simulink model "Lab4"  (R2025a)
settings: Solver=VariableStepAuto  StartTime=0.0  StopTime=20  RelTol=1e-3
settings Model: Creator=andrei  LastModifiedBy=andrei

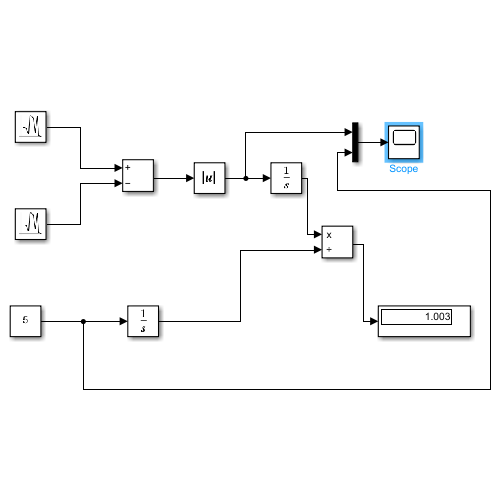
[thumbnail: Simulink's stored preview of the top-level diagram]
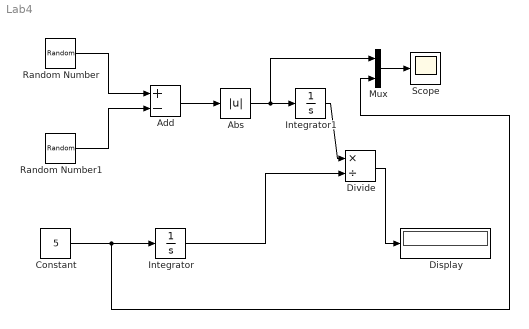
== system Lab4 ==
  Abs : Abs  SaturateOnIntegerOverflow=off
  Add : Sum  Inputs=+-
  Constant : Constant  Value=5
  Display : Display
  Divide : Product  Inputs=*/
  Integrator : Integrator
  Integrator1 : Integrator
  Mux : Mux  Inputs=2
  Random Number : RandomNumber  Mean=15  Variance=3  SampleTime=0.1
  Random Number1 : RandomNumber  Mean=10  Variance=2  SampleTime=0.1
  Scope : Scope
      settings: ActiveDisplayYMinimum=4.5698032026447679  ActiveDisplayYMaximum=5.6578783011741312
  wires:
  Random Number/1 -> Add/1
  Random Number1/1 -> Add/2
  Constant/1 -> Mux/2, Integrator/1
  Add/1 -> Abs/1
  Abs/1 -> Mux/1, Integrator1/1
  Integrator1/1 -> Divide/1
  Integrator/1 -> Divide/2
  Divide/1 -> Display/1
  Mux/1 -> Scope/1
